simulink model "regler_pi_mdl"  (R2013b)
settings: Solver=ode45  StartTime=0.0  StopTime=10.0  RelTol=1e-3
values from neighbouring files (symbols this model uses):
  K = 0.05    [regler_pi.m]
  Kg = K / (K*K + a*R)    (= 16.6666666667)    [regler_pi.m]
  Kp = 10    [regler_pi.m]
  mmax = 0.00    (= 0)    [regler_pi.m]
  R = 0.5    [regler_pi.m]
  tau = J*R / (K*K + a*R)    (= 0.0416666666667)    [regler_pi.m]
  Ti = tau    (= 0.0416666666667)    [regler_pi.m]
settings Model: Creator=daniw  LastModifiedBy=daniw
settings DataIOCC: LimitDataPoints=off

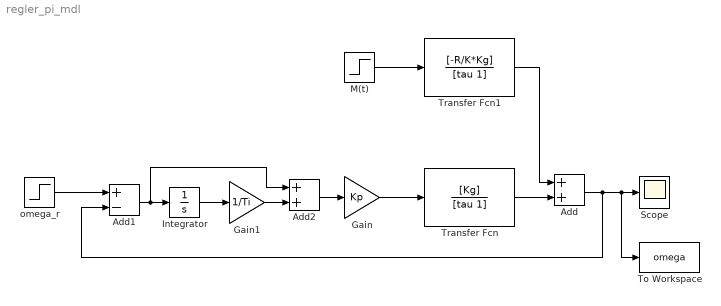
== system regler_pi_mdl ==
  Add : Sum
  Add1 : Sum  Inputs=+-
  Add2 : Sum
  Gain : Gain  Gain=Kp
  Gain1 : Gain  Gain=1/Ti
  Integrator : Integrator
  M(t) : Step  Time=2  After=mmax  SampleTime=0
  Scope : Scope
  To Workspace : ToWorkspace  VariableName=omega  SampleTime=-1  SaveFormat=Structure With Time
  Transfer Fcn : TransferFcn  Numerator=[Kg]  Denominator=[tau 1]
  Transfer Fcn1 : TransferFcn  Numerator=[-R/K*Kg]  Denominator=[tau 1]
  omega_r : Step  Before=5  After=20  SampleTime=0
  wires:
  M(t)/1 -> Transfer Fcn1/1
  omega_r/1 -> Add1/1
  Add/1 -> Add1/2, To Workspace/1, Scope/1
  Transfer Fcn/1 -> Add/2
  Transfer Fcn1/1 -> Add/1
  Gain/1 -> Transfer Fcn/1
  Add1/1 -> Add2/1, Integrator/1
  Integrator/1 -> Gain1/1
  Add2/1 -> Gain/1
  Gain1/1 -> Add2/2
